simulink model "orion_casestudy_16"  (R2023a)
settings: Solver=VariableStepAuto  StartTime=0.0  StopTime=30  RelTol=1e-3
InitFcn:
  | RandStream.setGlobalStream(RandStream('mt19937ar','seed',sum(100*clock)));
undefined symbols (not defined in the file or in its folder): m, n
(part 3 of 4)

== stateflow chart orion_casestudy_16/DelaySwitch129 ==
  state Operation
  state Sending
  (default) -> Operation : {i=0;}
  (junction 7) -> Operation [order 2]
  Sending -> Operation : after(delay_array(i),msec)
      | {receive(inMsg);outMsg.data=0;send(outMsg);}
  Operation -> (junction 7) : inMsg{i = i + 1;}
  (junction 7) -> Sending [order 1] : [switch_array(i)==0]
  data: switch_array input; delay_array input; outMsg output; inMsg input; i local

== stateflow chart orion_casestudy_16/DelaySwitch130 ==
  state Operation
  state Sending
  (default) -> Operation : {i=0;}
  (junction 7) -> Operation [order 2]
  Sending -> Operation : after(delay_array(i),msec)
      | {receive(inMsg);outMsg.data=0;send(outMsg);}
  Operation -> (junction 7) : inMsg{i = i + 1;}
  (junction 7) -> Sending [order 1] : [switch_array(i)==0]
  data: switch_array input; delay_array input; outMsg output; inMsg input; i local

== stateflow chart orion_casestudy_16/DelaySwitch131 ==
  state Operation
  state Sending
  (default) -> Operation : {i=0;}
  (junction 7) -> Operation [order 2]
  Sending -> Operation : after(delay_array(i),msec)
      | {receive(inMsg);outMsg.data=0;send(outMsg);}
  Operation -> (junction 7) : inMsg{i = i + 1;}
  (junction 7) -> Sending [order 1] : [switch_array(i)==0]
  data: switch_array input; delay_array input; outMsg output; inMsg input; i local

== stateflow chart orion_casestudy_16/DelaySwitch132 ==
  state Operation
  state Sending
  (default) -> Operation : {i=0;}
  (junction 7) -> Operation [order 2]
  Sending -> Operation : after(delay_array(i),msec)
      | {receive(inMsg);outMsg.data=0;send(outMsg);}
  Operation -> (junction 7) : inMsg{i = i + 1;}
  (junction 7) -> Sending [order 1] : [switch_array(i)==0]
  data: switch_array input; delay_array input; outMsg output; inMsg input; i local

== stateflow chart orion_casestudy_16/DelaySwitch133 ==
  state Operation
  state Sending
  (default) -> Operation : {i=0;}
  (junction 7) -> Operation [order 2]
  Sending -> Operation : after(delay_array(i),msec)
      | {receive(inMsg);outMsg.data=0;send(outMsg);}
  Operation -> (junction 7) : inMsg{i = i + 1;}
  (junction 7) -> Sending [order 1] : [switch_array(i)==0]
  data: switch_array input; delay_array input; outMsg output; inMsg input; i local

== stateflow chart orion_casestudy_16/DelaySwitch134 ==
  state Operation
  state Sending
  (default) -> Operation : {i=0;}
  (junction 7) -> Operation [order 2]
  Sending -> Operation : after(delay_array(i),msec)
      | {receive(inMsg);outMsg.data=0;send(outMsg);}
  Operation -> (junction 7) : inMsg{i = i + 1;}
  (junction 7) -> Sending [order 1] : [switch_array(i)==0]
  data: switch_array input; delay_array input; outMsg output; inMsg input; i local

== stateflow chart orion_casestudy_16/DelaySwitch135 ==
  state Operation
  state Sending
  (default) -> Operation : {i=0;}
  (junction 7) -> Operation [order 2]
  Sending -> Operation : after(delay_array(i),msec)
      | {receive(inMsg);outMsg.data=0;send(outMsg);}
  Operation -> (junction 7) : inMsg{i = i + 1;}
  (junction 7) -> Sending [order 1] : [switch_array(i)==0]
  data: switch_array input; delay_array input; outMsg output; inMsg input; i local

== stateflow chart orion_casestudy_16/DelaySwitch136 ==
  state Operation
  state Sending
  (default) -> Operation : {i=0;}
  (junction 7) -> Operation [order 2]
  Sending -> Operation : after(delay_array(i),msec)
      | {receive(inMsg);outMsg.data=0;send(outMsg);}
  Operation -> (junction 7) : inMsg{i = i + 1;}
  (junction 7) -> Sending [order 1] : [switch_array(i)==0]
  data: switch_array input; delay_array input; outMsg output; inMsg input; i local

== stateflow chart orion_casestudy_16/DelaySwitch137 ==
  state Operation
  state Sending
  (default) -> Operation : {i=0;}
  (junction 7) -> Operation [order 2]
  Sending -> Operation : after(delay_array(i),msec)
      | {receive(inMsg);outMsg.data=0;send(outMsg);}
  Operation -> (junction 7) : inMsg{i = i + 1;}
  (junction 7) -> Sending [order 1] : [switch_array(i)==0]
  data: switch_array input; delay_array input; outMsg output; inMsg input; i local

== stateflow chart orion_casestudy_16/DelaySwitch8 ==
  state Operation
  state Sending
  (default) -> Operation : {i=0;}
  (junction 7) -> Operation [order 2]
  Sending -> Operation : after(delay_array(i),msec)
      | {receive(inMsg);outMsg.data=0;send(outMsg);}
  Operation -> (junction 7) : inMsg{i = i + 1;}
  (junction 7) -> Sending [order 1] : [switch_array(i)==0]
  data: switch_array input; delay_array input; outMsg output; inMsg input; i local

== stateflow chart orion_casestudy_16/DelaySwitch138 ==
  state Operation
  state Sending
  (default) -> Operation : {i=0;}
  (junction 7) -> Operation [order 2]
  Sending -> Operation : after(delay_array(i),msec)
      | {receive(inMsg);outMsg.data=0;send(outMsg);}
  Operation -> (junction 7) : inMsg{i = i + 1;}
  (junction 7) -> Sending [order 1] : [switch_array(i)==0]
  data: switch_array input; delay_array input; outMsg output; inMsg input; i local

== stateflow chart orion_casestudy_16/DelaySwitch139 ==
  state Operation
  state Sending
  (default) -> Operation : {i=0;}
  (junction 7) -> Operation [order 2]
  Sending -> Operation : after(delay_array(i),msec)
      | {receive(inMsg);outMsg.data=0;send(outMsg);}
  Operation -> (junction 7) : inMsg{i = i + 1;}
  (junction 7) -> Sending [order 1] : [switch_array(i)==0]
  data: switch_array input; delay_array input; outMsg output; inMsg input; i local

== stateflow chart orion_casestudy_16/DelaySwitch140 ==
  state Operation
  state Sending
  (default) -> Operation : {i=0;}
  (junction 7) -> Operation [order 2]
  Sending -> Operation : after(delay_array(i),msec)
      | {receive(inMsg);outMsg.data=0;send(outMsg);}
  Operation -> (junction 7) : inMsg{i = i + 1;}
  (junction 7) -> Sending [order 1] : [switch_array(i)==0]
  data: switch_array input; delay_array input; outMsg output; inMsg input; i local

== stateflow chart orion_casestudy_16/DelaySwitch141 ==
  state Operation
  state Sending
  (default) -> Operation : {i=0;}
  (junction 7) -> Operation [order 2]
  Sending -> Operation : after(delay_array(i),msec)
      | {receive(inMsg);outMsg.data=0;send(outMsg);}
  Operation -> (junction 7) : inMsg{i = i + 1;}
  (junction 7) -> Sending [order 1] : [switch_array(i)==0]
  data: switch_array input; delay_array input; outMsg output; inMsg input; i local

== stateflow chart orion_casestudy_16/DelaySwitch142 ==
  state Operation
  state Sending
  (default) -> Operation : {i=0;}
  (junction 7) -> Operation [order 2]
  Sending -> Operation : after(delay_array(i),msec)
      | {receive(inMsg);outMsg.data=0;send(outMsg);}
  Operation -> (junction 7) : inMsg{i = i + 1;}
  (junction 7) -> Sending [order 1] : [switch_array(i)==0]
  data: switch_array input; delay_array input; outMsg output; inMsg input; i local

== stateflow chart orion_casestudy_16/DelaySwitch143 ==
  state Operation
  state Sending
  (default) -> Operation : {i=0;}
  (junction 7) -> Operation [order 2]
  Sending -> Operation : after(delay_array(i),msec)
      | {receive(inMsg);outMsg.data=0;send(outMsg);}
  Operation -> (junction 7) : inMsg{i = i + 1;}
  (junction 7) -> Sending [order 1] : [switch_array(i)==0]
  data: switch_array input; delay_array input; outMsg output; inMsg input; i local

== stateflow chart orion_casestudy_16/DelaySwitch144 ==
  state Operation
  state Sending
  (default) -> Operation : {i=0;}
  (junction 7) -> Operation [order 2]
  Sending -> Operation : after(delay_array(i),msec)
      | {receive(inMsg);outMsg.data=0;send(outMsg);}
  Operation -> (junction 7) : inMsg{i = i + 1;}
  (junction 7) -> Sending [order 1] : [switch_array(i)==0]
  data: switch_array input; delay_array input; outMsg output; inMsg input; i local

== stateflow chart orion_casestudy_16/DelaySwitch145 ==
  state Operation
  state Sending
  (default) -> Operation : {i=0;}
  (junction 7) -> Operation [order 2]
  Sending -> Operation : after(delay_array(i),msec)
      | {receive(inMsg);outMsg.data=0;send(outMsg);}
  Operation -> (junction 7) : inMsg{i = i + 1;}
  (junction 7) -> Sending [order 1] : [switch_array(i)==0]
  data: switch_array input; delay_array input; outMsg output; inMsg input; i local

== stateflow chart orion_casestudy_16/DelaySwitch146 ==
  state Operation
  state Sending
  (default) -> Operation : {i=0;}
  (junction 7) -> Operation [order 2]
  Sending -> Operation : after(delay_array(i),msec)
      | {receive(inMsg);outMsg.data=0;send(outMsg);}
  Operation -> (junction 7) : inMsg{i = i + 1;}
  (junction 7) -> Sending [order 1] : [switch_array(i)==0]
  data: switch_array input; delay_array input; outMsg output; inMsg input; i local

== stateflow chart orion_casestudy_16/DelaySwitch147 ==
  state Operation
  state Sending
  (default) -> Operation : {i=0;}
  (junction 7) -> Operation [order 2]
  Sending -> Operation : after(delay_array(i),msec)
      | {receive(inMsg);outMsg.data=0;send(outMsg);}
  Operation -> (junction 7) : inMsg{i = i + 1;}
  (junction 7) -> Sending [order 1] : [switch_array(i)==0]
  data: switch_array input; delay_array input; outMsg output; inMsg input; i local

== stateflow chart orion_casestudy_16/DelaySwitch9 ==
  state Operation
  state Sending
  (default) -> Operation : {i=0;}
  (junction 7) -> Operation [order 2]
  Sending -> Operation : after(delay_array(i),msec)
      | {receive(inMsg);outMsg.data=0;send(outMsg);}
  Operation -> (junction 7) : inMsg{i = i + 1;}
  (junction 7) -> Sending [order 1] : [switch_array(i)==0]
  data: switch_array input; delay_array input; outMsg output; inMsg input; i local

== stateflow chart orion_casestudy_16/DelaySwitch148 ==
  state Operation
  state Sending
  (default) -> Operation : {i=0;}
  (junction 7) -> Operation [order 2]
  Sending -> Operation : after(delay_array(i),msec)
      | {receive(inMsg);outMsg.data=0;send(outMsg);}
  Operation -> (junction 7) : inMsg{i = i + 1;}
  (junction 7) -> Sending [order 1] : [switch_array(i)==0]
  data: switch_array input; delay_array input; outMsg output; inMsg input; i local

== stateflow chart orion_casestudy_16/DelaySwitch149 ==
  state Operation
  state Sending
  (default) -> Operation : {i=0;}
  (junction 7) -> Operation [order 2]
  Sending -> Operation : after(delay_array(i),msec)
      | {receive(inMsg);outMsg.data=0;send(outMsg);}
  Operation -> (junction 7) : inMsg{i = i + 1;}
  (junction 7) -> Sending [order 1] : [switch_array(i)==0]
  data: switch_array input; delay_array input; outMsg output; inMsg input; i local

== stateflow chart orion_casestudy_16/DelaySwitch150 ==
  state Operation
  state Sending
  (default) -> Operation : {i=0;}
  (junction 7) -> Operation [order 2]
  Sending -> Operation : after(delay_array(i),msec)
      | {receive(inMsg);outMsg.data=0;send(outMsg);}
  Operation -> (junction 7) : inMsg{i = i + 1;}
  (junction 7) -> Sending [order 1] : [switch_array(i)==0]
  data: switch_array input; delay_array input; outMsg output; inMsg input; i local

== stateflow chart orion_casestudy_16/DelaySwitch151 ==
  state Operation
  state Sending
  (default) -> Operation : {i=0;}
  (junction 7) -> Operation [order 2]
  Sending -> Operation : after(delay_array(i),msec)
      | {receive(inMsg);outMsg.data=0;send(outMsg);}
  Operation -> (junction 7) : inMsg{i = i + 1;}
  (junction 7) -> Sending [order 1] : [switch_array(i)==0]
  data: switch_array input; delay_array input; outMsg output; inMsg input; i local

== stateflow chart orion_casestudy_16/DelaySwitch152 ==
  state Operation
  state Sending
  (default) -> Operation : {i=0;}
  (junction 7) -> Operation [order 2]
  Sending -> Operation : after(delay_array(i),msec)
      | {receive(inMsg);outMsg.data=0;send(outMsg);}
  Operation -> (junction 7) : inMsg{i = i + 1;}
  (junction 7) -> Sending [order 1] : [switch_array(i)==0]
  data: switch_array input; delay_array input; outMsg output; inMsg input; i local

== stateflow chart orion_casestudy_16/DelaySwitch153 ==
  state Operation
  state Sending
  (default) -> Operation : {i=0;}
  (junction 7) -> Operation [order 2]
  Sending -> Operation : after(delay_array(i),msec)
      | {receive(inMsg);outMsg.data=0;send(outMsg);}
  Operation -> (junction 7) : inMsg{i = i + 1;}
  (junction 7) -> Sending [order 1] : [switch_array(i)==0]
  data: switch_array input; delay_array input; outMsg output; inMsg input; i local

== stateflow chart orion_casestudy_16/DelaySwitch154 ==
  state Operation
  state Sending
  (default) -> Operation : {i=0;}
  (junction 7) -> Operation [order 2]
  Sending -> Operation : after(delay_array(i),msec)
      | {receive(inMsg);outMsg.data=0;send(outMsg);}
  Operation -> (junction 7) : inMsg{i = i + 1;}
  (junction 7) -> Sending [order 1] : [switch_array(i)==0]
  data: switch_array input; delay_array input; outMsg output; inMsg input; i local

== stateflow chart orion_casestudy_16/DelaySwitch155 ==
  state Operation
  state Sending
  (default) -> Operation : {i=0;}
  (junction 7) -> Operation [order 2]
  Sending -> Operation : after(delay_array(i),msec)
      | {receive(inMsg);outMsg.data=0;send(outMsg);}
  Operation -> (junction 7) : inMsg{i = i + 1;}
  (junction 7) -> Sending [order 1] : [switch_array(i)==0]
  data: switch_array input; delay_array input; outMsg output; inMsg input; i local

== stateflow chart orion_casestudy_16/DelaySwitch156 ==
  state Operation
  state Sending
  (default) -> Operation : {i=0;}
  (junction 7) -> Operation [order 2]
  Sending -> Operation : after(delay_array(i),msec)
      | {receive(inMsg);outMsg.data=0;send(outMsg);}
  Operation -> (junction 7) : inMsg{i = i + 1;}
  (junction 7) -> Sending [order 1] : [switch_array(i)==0]
  data: switch_array input; delay_array input; outMsg output; inMsg input; i local

== stateflow chart orion_casestudy_16/DelaySwitch157 ==
  state Operation
  state Sending
  (default) -> Operation : {i=0;}
  (junction 7) -> Operation [order 2]
  Sending -> Operation : after(delay_array(i),msec)
      | {receive(inMsg);outMsg.data=0;send(outMsg);}
  Operation -> (junction 7) : inMsg{i = i + 1;}
  (junction 7) -> Sending [order 1] : [switch_array(i)==0]
  data: switch_array input; delay_array input; outMsg output; inMsg input; i local

== stateflow chart orion_casestudy_16/DelaySwitch10 ==
  state Operation
  state Sending
  (default) -> Operation : {i=0;}
  (junction 7) -> Operation [order 2]
  Sending -> Operation : after(delay_array(i),msec)
      | {receive(inMsg);outMsg.data=0;send(outMsg);}
  Operation -> (junction 7) : inMsg{i = i + 1;}
  (junction 7) -> Sending [order 1] : [switch_array(i)==0]
  data: switch_array input; delay_array input; outMsg output; inMsg input; i local

== stateflow chart orion_casestudy_16/DelaySwitch158 ==
  state Operation
  state Sending
  (default) -> Operation : {i=0;}
  (junction 7) -> Operation [order 2]
  Sending -> Operation : after(delay_array(i),msec)
      | {receive(inMsg);outMsg.data=0;send(outMsg);}
  Operation -> (junction 7) : inMsg{i = i + 1;}
  (junction 7) -> Sending [order 1] : [switch_array(i)==0]
  data: switch_array input; delay_array input; outMsg output; inMsg input; i local

== stateflow chart orion_casestudy_16/DelaySwitch159 ==
  state Operation
  state Sending
  (default) -> Operation : {i=0;}
  (junction 7) -> Operation [order 2]
  Sending -> Operation : after(delay_array(i),msec)
      | {receive(inMsg);outMsg.data=0;send(outMsg);}
  Operation -> (junction 7) : inMsg{i = i + 1;}
  (junction 7) -> Sending [order 1] : [switch_array(i)==0]
  data: switch_array input; delay_array input; outMsg output; inMsg input; i local

== stateflow chart orion_casestudy_16/DelaySwitch160 ==
  state Operation
  state Sending
  (default) -> Operation : {i=0;}
  (junction 7) -> Operation [order 2]
  Sending -> Operation : after(delay_array(i),msec)
      | {receive(inMsg);outMsg.data=0;send(outMsg);}
  Operation -> (junction 7) : inMsg{i = i + 1;}
  (junction 7) -> Sending [order 1] : [switch_array(i)==0]
  data: switch_array input; delay_array input; outMsg output; inMsg input; i local

== stateflow chart orion_casestudy_16/DelaySwitch81 ==
  state Operation
  state Sending
  (default) -> Operation : {i=0;}
  (junction 7) -> Operation [order 2]
  Sending -> Operation : after(delay_array(i),msec)
      | {receive(inMsg);outMsg.data=0;send(outMsg);}
  Operation -> (junction 7) : inMsg{i = i + 1;}
  (junction 7) -> Sending [order 1] : [switch_array(i)==0]
  data: switch_array input; delay_array input; outMsg output; inMsg input; i local

== stateflow chart orion_casestudy_16/DelaySwitch82 ==
  state Operation
  state Sending
  (default) -> Operation : {i=0;}
  (junction 7) -> Operation [order 2]
  Sending -> Operation : after(delay_array(i),msec)
      | {receive(inMsg);outMsg.data=0;send(outMsg);}
  Operation -> (junction 7) : inMsg{i = i + 1;}
  (junction 7) -> Sending [order 1] : [switch_array(i)==0]
  data: switch_array input; delay_array input; outMsg output; inMsg input; i local

== stateflow chart orion_casestudy_16/DelaySwitch83 ==
  state Operation
  state Sending
  (default) -> Operation : {i=0;}
  (junction 7) -> Operation [order 2]
  Sending -> Operation : after(delay_array(i),msec)
      | {receive(inMsg);outMsg.data=0;send(outMsg);}
  Operation -> (junction 7) : inMsg{i = i + 1;}
  (junction 7) -> Sending [order 1] : [switch_array(i)==0]
  data: switch_array input; delay_array input; outMsg output; inMsg input; i local

== stateflow chart orion_casestudy_16/DelaySwitch84 ==
  state Operation
  state Sending
  (default) -> Operation : {i=0;}
  (junction 7) -> Operation [order 2]
  Sending -> Operation : after(delay_array(i),msec)
      | {receive(inMsg);outMsg.data=0;send(outMsg);}
  Operation -> (junction 7) : inMsg{i = i + 1;}
  (junction 7) -> Sending [order 1] : [switch_array(i)==0]
  data: switch_array input; delay_array input; outMsg output; inMsg input; i local

== stateflow chart orion_casestudy_16/DelaySwitch85 ==
  state Operation
  state Sending
  (default) -> Operation : {i=0;}
  (junction 7) -> Operation [order 2]
  Sending -> Operation : after(delay_array(i),msec)
      | {receive(inMsg);outMsg.data=0;send(outMsg);}
  Operation -> (junction 7) : inMsg{i = i + 1;}
  (junction 7) -> Sending [order 1] : [switch_array(i)==0]
  data: switch_array input; delay_array input; outMsg output; inMsg input; i local

== stateflow chart orion_casestudy_16/DelaySwitch86 ==
  state Operation
  state Sending
  (default) -> Operation : {i=0;}
  (junction 7) -> Operation [order 2]
  Sending -> Operation : after(delay_array(i),msec)
      | {receive(inMsg);outMsg.data=0;send(outMsg);}
  Operation -> (junction 7) : inMsg{i = i + 1;}
  (junction 7) -> Sending [order 1] : [switch_array(i)==0]
  data: switch_array input; delay_array input; outMsg output; inMsg input; i local

== stateflow chart orion_casestudy_16/DelaySwitch87 ==
  state Operation
  state Sending
  (default) -> Operation : {i=0;}
  (junction 7) -> Operation [order 2]
  Sending -> Operation : after(delay_array(i),msec)
      | {receive(inMsg);outMsg.data=0;send(outMsg);}
  Operation -> (junction 7) : inMsg{i = i + 1;}
  (junction 7) -> Sending [order 1] : [switch_array(i)==0]
  data: switch_array input; delay_array input; outMsg output; inMsg input; i local

== stateflow chart orion_casestudy_16/OverallState ==
  settings: updateMethod=CONTINUOUS
  state NotConnected
    op_time=temporalCount(msec);
  state Connected
    entry:
    connStatus=1;
  (default) -> NotConnected : {connStatus=0;
      | op_time=0;}
  NotConnected -> Connected : [(conn1==2 && conn2==2) ||  (conn3==2 && conn4==2) ||  (conn5==2 && conn6==2) ||  (conn7==2 && conn8==2) ||  (conn9==2 && conn10==2) ||  (conn11==2 && conn12==2) ||  (conn13==2 && conn14==2) ||  (conn15==2 && conn16==2) || (conn17==2 && conn18==2) ||  (conn19==2 && conn20==2) ||  (conn21==2 && conn22==2) ||  (conn23==2 && conn24==2) ||  (conn25==2 && conn26==2) ||  (conn27==2 && conn28==2) ||  (conn29==2 && conn30==2) ||  (conn31==2 && conn32==2)]
  data: conn32 input; conn26 input; conn23 input; conn1 input; conn2 input; connStatus output; op_time output; conn3 input; conn4 input; conn5 input; conn6 input; conn7 input; conn8 input; conn9 input; conn10 input; conn11 input; conn12 input; conn13 input; conn14 input; conn15 input; conn16 input; conn17 input; conn18 input; conn19 input; conn20 input; conn21 input; conn22 input; conn24 input; conn25 input; conn27 input; conn28 input; conn29 input; conn30 input; conn31 input

== stateflow chart orion_casestudy_16/DelaySwitch88 ==
  state Operation
  state Sending
  (default) -> Operation : {i=0;}
  (junction 7) -> Operation [order 2]
  Sending -> Operation : after(delay_array(i),msec)
      | {receive(inMsg);outMsg.data=0;send(outMsg);}
  Operation -> (junction 7) : inMsg{i = i + 1;}
  (junction 7) -> Sending [order 1] : [switch_array(i)==0]
  data: switch_array input; delay_array input; outMsg output; inMsg input; i local

== stateflow chart orion_casestudy_16/DelaySwitch89 ==
  state Operation
  state Sending
  (default) -> Operation : {i=0;}
  (junction 7) -> Operation [order 2]
  Sending -> Operation : after(delay_array(i),msec)
      | {receive(inMsg);outMsg.data=0;send(outMsg);}
  Operation -> (junction 7) : inMsg{i = i + 1;}
  (junction 7) -> Sending [order 1] : [switch_array(i)==0]
  data: switch_array input; delay_array input; outMsg output; inMsg input; i local

== stateflow chart orion_casestudy_16/DelaySwitch90 ==
  state Operation
  state Sending
  (default) -> Operation : {i=0;}
  (junction 7) -> Operation [order 2]
  Sending -> Operation : after(delay_array(i),msec)
      | {receive(inMsg);outMsg.data=0;send(outMsg);}
  Operation -> (junction 7) : inMsg{i = i + 1;}
  (junction 7) -> Sending [order 1] : [switch_array(i)==0]
  data: switch_array input; delay_array input; outMsg output; inMsg input; i local

== stateflow chart orion_casestudy_16/DelaySwitch91 ==
  state Operation
  state Sending
  (default) -> Operation : {i=0;}
  (junction 7) -> Operation [order 2]
  Sending -> Operation : after(delay_array(i),msec)
      | {receive(inMsg);outMsg.data=0;send(outMsg);}
  Operation -> (junction 7) : inMsg{i = i + 1;}
  (junction 7) -> Sending [order 1] : [switch_array(i)==0]
  data: switch_array input; delay_array input; outMsg output; inMsg input; i local

== stateflow chart orion_casestudy_16/DelaySwitch92 ==
  state Operation
  state Sending
  (default) -> Operation : {i=0;}
  (junction 7) -> Operation [order 2]
  Sending -> Operation : after(delay_array(i),msec)
      | {receive(inMsg);outMsg.data=0;send(outMsg);}
  Operation -> (junction 7) : inMsg{i = i + 1;}
  (junction 7) -> Sending [order 1] : [switch_array(i)==0]
  data: switch_array input; delay_array input; outMsg output; inMsg input; i local

== stateflow chart orion_casestudy_16/DelaySwitch93 ==
  state Operation
  state Sending
  (default) -> Operation : {i=0;}
  (junction 7) -> Operation [order 2]
  Sending -> Operation : after(delay_array(i),msec)
      | {receive(inMsg);outMsg.data=0;send(outMsg);}
  Operation -> (junction 7) : inMsg{i = i + 1;}
  (junction 7) -> Sending [order 1] : [switch_array(i)==0]
  data: switch_array input; delay_array input; outMsg output; inMsg input; i local

== stateflow chart orion_casestudy_16/DelaySwitch94 ==
  state Operation
  state Sending
  (default) -> Operation : {i=0;}
  (junction 7) -> Operation [order 2]
  Sending -> Operation : after(delay_array(i),msec)
      | {receive(inMsg);outMsg.data=0;send(outMsg);}
  Operation -> (junction 7) : inMsg{i = i + 1;}
  (junction 7) -> Sending [order 1] : [switch_array(i)==0]
  data: switch_array input; delay_array input; outMsg output; inMsg input; i local

== stateflow chart orion_casestudy_16/DelaySwitch95 ==
  state Operation
  state Sending
  (default) -> Operation : {i=0;}
  (junction 7) -> Operation [order 2]
  Sending -> Operation : after(delay_array(i),msec)
      | {receive(inMsg);outMsg.data=0;send(outMsg);}
  Operation -> (junction 7) : inMsg{i = i + 1;}
  (junction 7) -> Sending [order 1] : [switch_array(i)==0]
  data: switch_array input; delay_array input; outMsg output; inMsg input; i local

== stateflow chart orion_casestudy_16/DelaySwitch96 ==
  state Operation
  state Sending
  (default) -> Operation : {i=0;}
  (junction 7) -> Operation [order 2]
  Sending -> Operation : after(delay_array(i),msec)
      | {receive(inMsg);outMsg.data=0;send(outMsg);}
  Operation -> (junction 7) : inMsg{i = i + 1;}
  (junction 7) -> Sending [order 1] : [switch_array(i)==0]
  data: switch_array input; delay_array input; outMsg output; inMsg input; i local

== stateflow chart orion_casestudy_16/DelaySwitch97 ==
  state Operation
  state Sending
  (default) -> Operation : {i=0;}
  (junction 7) -> Operation [order 2]
  Sending -> Operation : after(delay_array(i),msec)
      | {receive(inMsg);outMsg.data=0;send(outMsg);}
  Operation -> (junction 7) : inMsg{i = i + 1;}
  (junction 7) -> Sending [order 1] : [switch_array(i)==0]
  data: switch_array input; delay_array input; outMsg output; inMsg input; i local

== stateflow chart orion_casestudy_16/DelaySwitch98 ==
  state Operation
  state Sending
  (default) -> Operation : {i=0;}
  (junction 7) -> Operation [order 2]
  Sending -> Operation : after(delay_array(i),msec)
      | {receive(inMsg);outMsg.data=0;send(outMsg);}
  Operation -> (junction 7) : inMsg{i = i + 1;}
  (junction 7) -> Sending [order 1] : [switch_array(i)==0]
  data: switch_array input; delay_array input; outMsg output; inMsg input; i local

== stateflow chart orion_casestudy_16/DelaySwitch99 ==
  state Operation
  state Sending
  (default) -> Operation : {i=0;}
  (junction 7) -> Operation [order 2]
  Sending -> Operation : after(delay_array(i),msec)
      | {receive(inMsg);outMsg.data=0;send(outMsg);}
  Operation -> (junction 7) : inMsg{i = i + 1;}
  (junction 7) -> Sending [order 1] : [switch_array(i)==0]
  data: switch_array input; delay_array input; outMsg output; inMsg input; i local

== stateflow chart orion_casestudy_16/Master10 ==
  settings: updateMethod=CONTINUOUS
  state Connected
    entry:
    connStatus=2;
    state KeepAliveSendTimeout [parallel]
      settings: executionOrder=1
      state KeepAliveSend
      (default) -> KeepAliveSend
      KeepAliveSend -> KeepAliveSend [order 1] : after(delay_array(i)*5,msec)
          | {OrionKeepAliveOut.data=0;
          | send(OrionKeepAliveOut);
          | i = i + 1;}
      KeepAliveSend -> KeepAliveSend [order 2] : SendDataIn
          | {OrionAppDataOut.data=0;
          | send(OrionAppDataOut);}
    state KeepAliveRecieveTimeout [parallel]
      settings: executionOrder=2
      state KeepAlineRec
      (default) -> KeepAlineRec
      KeepAlineRec -> KeepAlineRec [order 2] : OrionKeepAliveIn
      KeepAlineRec -> KeepAlineRec [order 3] : OrionAppDataIn
  state Closed
    entry:
    connStatus=0;
  state Connecting
    entry:
    connStatus=1;
  Connected -> (junction 6) [order 1] : OrionConnConfIn
  (default) -> Closed : {i=1;}
  Connected -> (junction 6) [order 2] : OrionConnRespIn
  Connected -> (junction 6) [order 3] : OrionConnReqIn
  (junction 6) -> Closed
  KeepAlineRec -> Closed [order 1] : after(delay_array(i)*5,msec)
      | {i = i + 1;}
  Connecting -> (junction 36) [order 5] : OrionConnReqIn
  (junction 36) -> Closed
  Connecting -> (junction 36) [order 4] : OrionConnRespIn
  Connecting -> (junction 36) [order 2] : OrionKeepAliveIn
  Connecting -> Closed [order 3] : after(delay_array(i)*5,msec)
      | {i = i + 1;}
  Closed -> Connecting [order 2] : after(delay_array(i)*5,msec)
      | {OrionConnReqOut.data=0;send(OrionConnReqOut);i = i + 1;}
  Closed -> Connecting [order 1] : OrionConnReqIn
      | {OrionConnRespOut.data=0;send(OrionConnRespOut);}
  Connecting -> Connected [order 1] : OrionConnRespIn
      | {OrionConnConfOut.data=0;
      | send(OrionConnConfOut);}
  data: delay_array input; OrionKeepAliveOut output; OrionKeepAliveIn input; OrionConnConfOut output; OrionConnConfIn input; OrionConnRespOut output; OrionAppDataOut output; OrionAppDataIn input; OrionConnRespIn input; OrionConnReqIn input; OrionConnReqOut output; connStatus output; SendDataIn local; i local

== stateflow chart orion_casestudy_16/Master11 ==
  settings: updateMethod=CONTINUOUS
  state Connected
    entry:
    connStatus=2;
    state KeepAliveSendTimeout [parallel]
      settings: executionOrder=1
      state KeepAliveSend
      (default) -> KeepAliveSend
      KeepAliveSend -> KeepAliveSend [order 1] : after(delay_array(i)*5,msec)
          | {OrionKeepAliveOut.data=0;
          | send(OrionKeepAliveOut);
          | i = i + 1;}
      KeepAliveSend -> KeepAliveSend [order 2] : SendDataIn
          | {OrionAppDataOut.data=0;
          | send(OrionAppDataOut);}
    state KeepAliveRecieveTimeout [parallel]
      settings: executionOrder=2
      state KeepAlineRec
      (default) -> KeepAlineRec
      KeepAlineRec -> KeepAlineRec [order 2] : OrionKeepAliveIn
      KeepAlineRec -> KeepAlineRec [order 3] : OrionAppDataIn
  state Closed
    entry:
    connStatus=0;
  state Connecting
    entry:
    connStatus=1;
  Connected -> (junction 6) [order 1] : OrionConnConfIn
  (default) -> Closed : {i=1;}
  Connected -> (junction 6) [order 2] : OrionConnRespIn
  Connected -> (junction 6) [order 3] : OrionConnReqIn
  (junction 6) -> Closed
  KeepAlineRec -> Closed [order 1] : after(delay_array(i)*5,msec)
      | {i = i + 1;}
  Connecting -> (junction 36) [order 5] : OrionConnReqIn
  (junction 36) -> Closed
  Connecting -> (junction 36) [order 4] : OrionConnRespIn
  Connecting -> (junction 36) [order 2] : OrionKeepAliveIn
  Connecting -> Closed [order 3] : after(delay_array(i)*5,msec)
      | {i = i + 1;}
  Closed -> Connecting [order 2] : after(delay_array(i)*5,msec)
      | {OrionConnReqOut.data=0;send(OrionConnReqOut);i = i + 1;}
  Closed -> Connecting [order 1] : OrionConnReqIn
      | {OrionConnRespOut.data=0;send(OrionConnRespOut);}
  Connecting -> Connected [order 1] : OrionConnRespIn
      | {OrionConnConfOut.data=0;
      | send(OrionConnConfOut);}
  data: delay_array input; OrionKeepAliveOut output; OrionKeepAliveIn input; OrionConnConfOut output; OrionConnConfIn input; OrionConnRespOut output; OrionAppDataOut output; OrionAppDataIn input; OrionConnRespIn input; OrionConnReqIn input; OrionConnReqOut output; connStatus output; SendDataIn local; i local

== stateflow chart orion_casestudy_16/Master12 ==
  settings: updateMethod=CONTINUOUS
  state Connected
    entry:
    connStatus=2;
    state KeepAliveSendTimeout [parallel]
      settings: executionOrder=1
      state KeepAliveSend
      (default) -> KeepAliveSend
      KeepAliveSend -> KeepAliveSend [order 1] : after(delay_array(i)*5,msec)
          | {OrionKeepAliveOut.data=0;
          | send(OrionKeepAliveOut);
          | i = i + 1;}
      KeepAliveSend -> KeepAliveSend [order 2] : SendDataIn
          | {OrionAppDataOut.data=0;
          | send(OrionAppDataOut);}
    state KeepAliveRecieveTimeout [parallel]
      settings: executionOrder=2
      state KeepAlineRec
      (default) -> KeepAlineRec
      KeepAlineRec -> KeepAlineRec [order 2] : OrionKeepAliveIn
      KeepAlineRec -> KeepAlineRec [order 3] : OrionAppDataIn
  state Closed
    entry:
    connStatus=0;
  state Connecting
    entry:
    connStatus=1;
  Connected -> (junction 6) [order 1] : OrionConnConfIn
  (default) -> Closed : {i=1;}
  Connected -> (junction 6) [order 2] : OrionConnRespIn
  Connected -> (junction 6) [order 3] : OrionConnReqIn
  (junction 6) -> Closed
  KeepAlineRec -> Closed [order 1] : after(delay_array(i)*5,msec)
      | {i = i + 1;}
  Connecting -> (junction 36) [order 5] : OrionConnReqIn
  (junction 36) -> Closed
  Connecting -> (junction 36) [order 4] : OrionConnRespIn
  Connecting -> (junction 36) [order 2] : OrionKeepAliveIn
  Connecting -> Closed [order 3] : after(delay_array(i)*5,msec)
      | {i = i + 1;}
  Closed -> Connecting [order 2] : after(delay_array(i)*5,msec)
      | {OrionConnReqOut.data=0;send(OrionConnReqOut);i = i + 1;}
  Closed -> Connecting [order 1] : OrionConnReqIn
      | {OrionConnRespOut.data=0;send(OrionConnRespOut);}
  Connecting -> Connected [order 1] : OrionConnRespIn
      | {OrionConnConfOut.data=0;
      | send(OrionConnConfOut);}
  data: delay_array input; OrionKeepAliveOut output; OrionKeepAliveIn input; OrionConnConfOut output; OrionConnConfIn input; OrionConnRespOut output; OrionAppDataOut output; OrionAppDataIn input; OrionConnRespIn input; OrionConnReqIn input; OrionConnReqOut output; connStatus output; SendDataIn local; i local

== stateflow chart orion_casestudy_16/Master13 ==
  settings: updateMethod=CONTINUOUS
  state Connected
    entry:
    connStatus=2;
    state KeepAliveSendTimeout [parallel]
      settings: executionOrder=1
      state KeepAliveSend
      (default) -> KeepAliveSend
      KeepAliveSend -> KeepAliveSend [order 1] : after(delay_array(i)*5,msec)
          | {OrionKeepAliveOut.data=0;
          | send(OrionKeepAliveOut);
          | i = i + 1;}
      KeepAliveSend -> KeepAliveSend [order 2] : SendDataIn
          | {OrionAppDataOut.data=0;
          | send(OrionAppDataOut);}
    state KeepAliveRecieveTimeout [parallel]
      settings: executionOrder=2
      state KeepAlineRec
      (default) -> KeepAlineRec
      KeepAlineRec -> KeepAlineRec [order 2] : OrionKeepAliveIn
      KeepAlineRec -> KeepAlineRec [order 3] : OrionAppDataIn
  state Closed
    entry:
    connStatus=0;
  state Connecting
    entry:
    connStatus=1;
  Connected -> (junction 6) [order 1] : OrionConnConfIn
  (default) -> Closed : {i=1;}
  Connected -> (junction 6) [order 2] : OrionConnRespIn
  Connected -> (junction 6) [order 3] : OrionConnReqIn
  (junction 6) -> Closed
  KeepAlineRec -> Closed [order 1] : after(delay_array(i)*5,msec)
      | {i = i + 1;}
  Connecting -> (junction 36) [order 5] : OrionConnReqIn
  (junction 36) -> Closed
  Connecting -> (junction 36) [order 4] : OrionConnRespIn
  Connecting -> (junction 36) [order 2] : OrionKeepAliveIn
  Connecting -> Closed [order 3] : after(delay_array(i)*5,msec)
      | {i = i + 1;}
  Closed -> Connecting [order 2] : after(delay_array(i)*5,msec)
      | {OrionConnReqOut.data=0;send(OrionConnReqOut);i = i + 1;}
  Closed -> Connecting [order 1] : OrionConnReqIn
      | {OrionConnRespOut.data=0;send(OrionConnRespOut);}
  Connecting -> Connected [order 1] : OrionConnRespIn
      | {OrionConnConfOut.data=0;
      | send(OrionConnConfOut);}
  data: delay_array input; OrionKeepAliveOut output; OrionKeepAliveIn input; OrionConnConfOut output; OrionConnConfIn input; OrionConnRespOut output; OrionAppDataOut output; OrionAppDataIn input; OrionConnRespIn input; OrionConnReqIn input; OrionConnReqOut output; connStatus output; SendDataIn local; i local

== stateflow chart orion_casestudy_16/Master14 ==
  settings: updateMethod=CONTINUOUS
  state Connected
    entry:
    connStatus=2;
    state KeepAliveSendTimeout [parallel]
      settings: executionOrder=1
      state KeepAliveSend
      (default) -> KeepAliveSend
      KeepAliveSend -> KeepAliveSend [order 1] : after(delay_array(i)*5,msec)
          | {OrionKeepAliveOut.data=0;
          | send(OrionKeepAliveOut);
          | i = i + 1;}
      KeepAliveSend -> KeepAliveSend [order 2] : SendDataIn
          | {OrionAppDataOut.data=0;
          | send(OrionAppDataOut);}
    state KeepAliveRecieveTimeout [parallel]
      settings: executionOrder=2
      state KeepAlineRec
      (default) -> KeepAlineRec
      KeepAlineRec -> KeepAlineRec [order 2] : OrionKeepAliveIn
      KeepAlineRec -> KeepAlineRec [order 3] : OrionAppDataIn
  state Closed
    entry:
    connStatus=0;
  state Connecting
    entry:
    connStatus=1;
  Connected -> (junction 6) [order 1] : OrionConnConfIn
  (default) -> Closed : {i=1;}
  Connected -> (junction 6) [order 2] : OrionConnRespIn
  Connected -> (junction 6) [order 3] : OrionConnReqIn
  (junction 6) -> Closed
  KeepAlineRec -> Closed [order 1] : after(delay_array(i)*5,msec)
      | {i = i + 1;}
  Connecting -> (junction 36) [order 5] : OrionConnReqIn
  (junction 36) -> Closed
  Connecting -> (junction 36) [order 4] : OrionConnRespIn
  Connecting -> (junction 36) [order 2] : OrionKeepAliveIn
  Connecting -> Closed [order 3] : after(delay_array(i)*5,msec)
      | {i = i + 1;}
  Closed -> Connecting [order 2] : after(delay_array(i)*5,msec)
      | {OrionConnReqOut.data=0;send(OrionConnReqOut);i = i + 1;}
  Closed -> Connecting [order 1] : OrionConnReqIn
      | {OrionConnRespOut.data=0;send(OrionConnRespOut);}
  Connecting -> Connected [order 1] : OrionConnRespIn
      | {OrionConnConfOut.data=0;
      | send(OrionConnConfOut);}
  data: delay_array input; OrionKeepAliveOut output; OrionKeepAliveIn input; OrionConnConfOut output; OrionConnConfIn input; OrionConnRespOut output; OrionAppDataOut output; OrionAppDataIn input; OrionConnRespIn input; OrionConnReqIn input; OrionConnReqOut output; connStatus output; SendDataIn local; i local

== stateflow chart orion_casestudy_16/DelaySwitch11 ==
  state Operation
  state Sending
  (default) -> Operation : {i=0;}
  (junction 7) -> Operation [order 2]
  Sending -> Operation : after(delay_array(i),msec)
      | {receive(inMsg);outMsg.data=0;send(outMsg);}
  Operation -> (junction 7) : inMsg{i = i + 1;}
  (junction 7) -> Sending [order 1] : [switch_array(i)==0]
  data: switch_array input; delay_array input; outMsg output; inMsg input; i local

== stateflow chart orion_casestudy_16/Master15 ==
  settings: updateMethod=CONTINUOUS
  state Connected
    entry:
    connStatus=2;
    state KeepAliveSendTimeout [parallel]
      settings: executionOrder=1
      state KeepAliveSend
      (default) -> KeepAliveSend
      KeepAliveSend -> KeepAliveSend [order 1] : after(delay_array(i)*5,msec)
          | {OrionKeepAliveOut.data=0;
          | send(OrionKeepAliveOut);
          | i = i + 1;}
      KeepAliveSend -> KeepAliveSend [order 2] : SendDataIn
          | {OrionAppDataOut.data=0;
          | send(OrionAppDataOut);}
    state KeepAliveRecieveTimeout [parallel]
      settings: executionOrder=2
      state KeepAlineRec
      (default) -> KeepAlineRec
      KeepAlineRec -> KeepAlineRec [order 2] : OrionKeepAliveIn
      KeepAlineRec -> KeepAlineRec [order 3] : OrionAppDataIn
  state Closed
    entry:
    connStatus=0;
  state Connecting
    entry:
    connStatus=1;
  Connected -> (junction 6) [order 1] : OrionConnConfIn
  (default) -> Closed : {i=1;}
  Connected -> (junction 6) [order 2] : OrionConnRespIn
  Connected -> (junction 6) [order 3] : OrionConnReqIn
  (junction 6) -> Closed
  KeepAlineRec -> Closed [order 1] : after(delay_array(i)*5,msec)
      | {i = i + 1;}
  Connecting -> (junction 36) [order 5] : OrionConnReqIn
  (junction 36) -> Closed
  Connecting -> (junction 36) [order 4] : OrionConnRespIn
  Connecting -> (junction 36) [order 2] : OrionKeepAliveIn
  Connecting -> Closed [order 3] : after(delay_array(i)*5,msec)
      | {i = i + 1;}
  Closed -> Connecting [order 2] : after(delay_array(i)*5,msec)
      | {OrionConnReqOut.data=0;send(OrionConnReqOut);i = i + 1;}
  Closed -> Connecting [order 1] : OrionConnReqIn
      | {OrionConnRespOut.data=0;send(OrionConnRespOut);}
  Connecting -> Connected [order 1] : OrionConnRespIn
      | {OrionConnConfOut.data=0;
      | send(OrionConnConfOut);}
  data: delay_array input; OrionKeepAliveOut output; OrionKeepAliveIn input; OrionConnConfOut output; OrionConnConfIn input; OrionConnRespOut output; OrionAppDataOut output; OrionAppDataIn input; OrionConnRespIn input; OrionConnReqIn input; OrionConnReqOut output; connStatus output; SendDataIn local; i local

== stateflow chart orion_casestudy_16/Master8 ==
  settings: updateMethod=CONTINUOUS
  state Connected
    entry:
    connStatus=2;
    state KeepAliveSendTimeout [parallel]
      settings: executionOrder=1
      state KeepAliveSend
      (default) -> KeepAliveSend
      KeepAliveSend -> KeepAliveSend [order 1] : after(delay_array(i)*5,msec)
          | {OrionKeepAliveOut.data=0;
          | send(OrionKeepAliveOut);
          | i = i + 1;}
      KeepAliveSend -> KeepAliveSend [order 2] : SendDataIn
          | {OrionAppDataOut.data=0;
          | send(OrionAppDataOut);}
    state KeepAliveRecieveTimeout [parallel]
      settings: executionOrder=2
      state KeepAlineRec
      (default) -> KeepAlineRec
      KeepAlineRec -> KeepAlineRec [order 2] : OrionKeepAliveIn
      KeepAlineRec -> KeepAlineRec [order 3] : OrionAppDataIn
  state Closed
    entry:
    connStatus=0;
  state Connecting
    entry:
    connStatus=1;
  Connected -> (junction 6) [order 1] : OrionConnConfIn
  (default) -> Closed : {i=1;}
  Connected -> (junction 6) [order 2] : OrionConnRespIn
  Connected -> (junction 6) [order 3] : OrionConnReqIn
  (junction 6) -> Closed
  KeepAlineRec -> Closed [order 1] : after(delay_array(i)*5,msec)
      | {i = i + 1;}
  Connecting -> (junction 36) [order 5] : OrionConnReqIn
  (junction 36) -> Closed
  Connecting -> (junction 36) [order 4] : OrionConnRespIn
  Connecting -> (junction 36) [order 2] : OrionKeepAliveIn
  Connecting -> Closed [order 3] : after(delay_array(i)*5,msec)
      | {i = i + 1;}
  Closed -> Connecting [order 2] : after(delay_array(i)*5,msec)
      | {OrionConnReqOut.data=0;send(OrionConnReqOut);i = i + 1;}
  Closed -> Connecting [order 1] : OrionConnReqIn
      | {OrionConnRespOut.data=0;send(OrionConnRespOut);}
  Connecting -> Connected [order 1] : OrionConnRespIn
      | {OrionConnConfOut.data=0;
      | send(OrionConnConfOut);}
  data: delay_array input; OrionKeepAliveOut output; OrionKeepAliveIn input; OrionConnConfOut output; OrionConnConfIn input; OrionConnRespOut output; OrionAppDataOut output; OrionAppDataIn input; OrionConnRespIn input; OrionConnReqIn input; OrionConnReqOut output; connStatus output; SendDataIn local; i local

== stateflow chart orion_casestudy_16/Master9 ==
  settings: updateMethod=CONTINUOUS
  state Connected
    entry:
    connStatus=2;
    state KeepAliveSendTimeout [parallel]
      settings: executionOrder=1
      state KeepAliveSend
      (default) -> KeepAliveSend
      KeepAliveSend -> KeepAliveSend [order 1] : after(delay_array(i)*5,msec)
          | {OrionKeepAliveOut.data=0;
          | send(OrionKeepAliveOut);
          | i = i + 1;}
      KeepAliveSend -> KeepAliveSend [order 2] : SendDataIn
          | {OrionAppDataOut.data=0;
          | send(OrionAppDataOut);}
    state KeepAliveRecieveTimeout [parallel]
      settings: executionOrder=2
      state KeepAlineRec
      (default) -> KeepAlineRec
      KeepAlineRec -> KeepAlineRec [order 2] : OrionKeepAliveIn
      KeepAlineRec -> KeepAlineRec [order 3] : OrionAppDataIn
  state Closed
    entry:
    connStatus=0;
  state Connecting
    entry:
    connStatus=1;
  Connected -> (junction 6) [order 1] : OrionConnConfIn
  (default) -> Closed : {i=1;}
  Connected -> (junction 6) [order 2] : OrionConnRespIn
  Connected -> (junction 6) [order 3] : OrionConnReqIn
  (junction 6) -> Closed
  KeepAlineRec -> Closed [order 1] : after(delay_array(i)*5,msec)
      | {i = i + 1;}
  Connecting -> (junction 36) [order 5] : OrionConnReqIn
  (junction 36) -> Closed
  Connecting -> (junction 36) [order 4] : OrionConnRespIn
  Connecting -> (junction 36) [order 2] : OrionKeepAliveIn
  Connecting -> Closed [order 3] : after(delay_array(i)*5,msec)
      | {i = i + 1;}
  Closed -> Connecting [order 2] : after(delay_array(i)*5,msec)
      | {OrionConnReqOut.data=0;send(OrionConnReqOut);i = i + 1;}
  Closed -> Connecting [order 1] : OrionConnReqIn
      | {OrionConnRespOut.data=0;send(OrionConnRespOut);}
  Connecting -> Connected [order 1] : OrionConnRespIn
      | {OrionConnConfOut.data=0;
      | send(OrionConnConfOut);}
  data: delay_array input; OrionKeepAliveOut output; OrionKeepAliveIn input; OrionConnConfOut output; OrionConnConfIn input; OrionConnRespOut output; OrionAppDataOut output; OrionAppDataIn input; OrionConnRespIn input; OrionConnReqIn input; OrionConnReqOut output; connStatus output; SendDataIn local; i local

== stateflow chart orion_casestudy_16/DelaySwitch12 ==
  state Operation
  state Sending
  (default) -> Operation : {i=0;}
  (junction 7) -> Operation [order 2]
  Sending -> Operation : after(delay_array(i),msec)
      | {receive(inMsg);outMsg.data=0;send(outMsg);}
  Operation -> (junction 7) : inMsg{i = i + 1;}
  (junction 7) -> Sending [order 1] : [switch_array(i)==0]
  data: switch_array input; delay_array input; outMsg output; inMsg input; i local

== stateflow chart orion_casestudy_16/Slave10 ==
  settings: updateMethod=CONTINUOUS
  state Connected
    entry:
    connStatus=2;
    state KeepAliveSendTimeout [parallel]
      settings: executionOrder=1
      state KeepAliveSend
      (default) -> KeepAliveSend
      KeepAliveSend -> KeepAliveSend [order 1] : after(delay_array(i)*5,msec)
          |  {OrionKeepAliveOut.data=0;
          | send(OrionKeepAliveOut);i = i + 1;}
      KeepAliveSend -> KeepAliveSend [order 2] : SendDataIn
          | {OrionAppDataOut.data=0;
          | send(OrionAppDataOut);}
    state KeepAliveRecieveTimeout [parallel]
      settings: executionOrder=2
      state KeepAlineRec
      (default) -> KeepAlineRec
      KeepAlineRec -> KeepAlineRec [order 2] : OrionKeepAliveIn
      KeepAlineRec -> KeepAlineRec [order 3] : OrionAppDataIn
  state Closed
    entry:
    connStatus=0;
  state Connecting
    entry:
    connStatus=1;
  Connected -> (junction 6) [order 2] : OrionConnRespIn
  Connected -> (junction 6) [order 3] : OrionConnReqIn
  (default) -> Closed : {i=1;}
  (junction 6) -> Closed
  Connected -> (junction 6) [order 1] : OrionConnConfIn
  KeepAlineRec -> Closed [order 1] : after(delay_array(i)*5,msec)
      | {i = i + 1;}
  Connecting -> (junction 36) [order 6] : OrionAppDataIn
  Connecting -> (junction 36) [order 5] : OrionConnReqIn
  (junction 36) -> Closed
  Connecting -> (junction 36) [order 4] : OrionConnRespIn
  Connecting -> (junction 36) [order 3] : OrionKeepAliveIn
  Closed -> Connecting : OrionConnReqIn
      | {OrionConnRespOut.data=0;
      | send(OrionConnRespOut);}
  Connecting -> Closed [order 1] : after(delay_array(i)*5,msec)
      | {i = i + 1;}
  Connecting -> Connected [order 2] : OrionConnConfIn{OrionConnConfOut.data=0;send(OrionConnConfOut);}
  data: OrionKeepAliveIn input; OrionConnConfOut output; OrionConnRespOut output; OrionKeepAliveOut output; OrionAppDataOut output; OrionAppDataIn input; OrionConnRespIn input; OrionConnReqIn input; OrionConnReqOut output size=1; connStatus output; SendDataIn local; OrionConnConfIn input; delay_array input; i local

== stateflow chart orion_casestudy_16/Slave11 ==
  settings: updateMethod=CONTINUOUS
  state Connected
    entry:
    connStatus=2;
    state KeepAliveSendTimeout [parallel]
      settings: executionOrder=1
      state KeepAliveSend
      (default) -> KeepAliveSend
      KeepAliveSend -> KeepAliveSend [order 1] : after(delay_array(i)*5,msec)
          |  {OrionKeepAliveOut.data=0;
          | send(OrionKeepAliveOut);i = i + 1;}
      KeepAliveSend -> KeepAliveSend [order 2] : SendDataIn
          | {OrionAppDataOut.data=0;
          | send(OrionAppDataOut);}
    state KeepAliveRecieveTimeout [parallel]
      settings: executionOrder=2
      state KeepAlineRec
      (default) -> KeepAlineRec
      KeepAlineRec -> KeepAlineRec [order 2] : OrionKeepAliveIn
      KeepAlineRec -> KeepAlineRec [order 3] : OrionAppDataIn
  state Closed
    entry:
    connStatus=0;
  state Connecting
    entry:
    connStatus=1;
  Connected -> (junction 6) [order 2] : OrionConnRespIn
  Connected -> (junction 6) [order 3] : OrionConnReqIn
  (default) -> Closed : {i=1;}
  (junction 6) -> Closed
  Connected -> (junction 6) [order 1] : OrionConnConfIn
  KeepAlineRec -> Closed [order 1] : after(delay_array(i)*5,msec)
      | {i = i + 1;}
  Connecting -> (junction 36) [order 6] : OrionAppDataIn
  Connecting -> (junction 36) [order 5] : OrionConnReqIn
  (junction 36) -> Closed
  Connecting -> (junction 36) [order 4] : OrionConnRespIn
  Connecting -> (junction 36) [order 3] : OrionKeepAliveIn
  Closed -> Connecting : OrionConnReqIn
      | {OrionConnRespOut.data=0;
      | send(OrionConnRespOut);}
  Connecting -> Closed [order 1] : after(delay_array(i)*5,msec)
      | {i = i + 1;}
  Connecting -> Connected [order 2] : OrionConnConfIn{OrionConnConfOut.data=0;send(OrionConnConfOut);}
  data: OrionKeepAliveIn input; OrionConnConfOut output; OrionConnRespOut output; OrionKeepAliveOut output; OrionAppDataOut output; OrionAppDataIn input; OrionConnRespIn input; OrionConnReqIn input; OrionConnReqOut output size=1; connStatus output; SendDataIn local; OrionConnConfIn input; delay_array input; i local

== stateflow chart orion_casestudy_16/Slave12 ==
  settings: updateMethod=CONTINUOUS
  state Connected
    entry:
    connStatus=2;
    state KeepAliveSendTimeout [parallel]
      settings: executionOrder=1
      state KeepAliveSend
      (default) -> KeepAliveSend
      KeepAliveSend -> KeepAliveSend [order 1] : after(delay_array(i)*5,msec)
          |  {OrionKeepAliveOut.data=0;
          | send(OrionKeepAliveOut);i = i + 1;}
      KeepAliveSend -> KeepAliveSend [order 2] : SendDataIn
          | {OrionAppDataOut.data=0;
          | send(OrionAppDataOut);}
    state KeepAliveRecieveTimeout [parallel]
      settings: executionOrder=2
      state KeepAlineRec
      (default) -> KeepAlineRec
      KeepAlineRec -> KeepAlineRec [order 2] : OrionKeepAliveIn
      KeepAlineRec -> KeepAlineRec [order 3] : OrionAppDataIn
  state Closed
    entry:
    connStatus=0;
  state Connecting
    entry:
    connStatus=1;
  Connected -> (junction 6) [order 2] : OrionConnRespIn
  Connected -> (junction 6) [order 3] : OrionConnReqIn
  (default) -> Closed : {i=1;}
  (junction 6) -> Closed
  Connected -> (junction 6) [order 1] : OrionConnConfIn
  KeepAlineRec -> Closed [order 1] : after(delay_array(i)*5,msec)
      | {i = i + 1;}
  Connecting -> (junction 36) [order 6] : OrionAppDataIn
  Connecting -> (junction 36) [order 5] : OrionConnReqIn
  (junction 36) -> Closed
  Connecting -> (junction 36) [order 4] : OrionConnRespIn
  Connecting -> (junction 36) [order 3] : OrionKeepAliveIn
  Closed -> Connecting : OrionConnReqIn
      | {OrionConnRespOut.data=0;
      | send(OrionConnRespOut);}
  Connecting -> Closed [order 1] : after(delay_array(i)*5,msec)
      | {i = i + 1;}
  Connecting -> Connected [order 2] : OrionConnConfIn{OrionConnConfOut.data=0;send(OrionConnConfOut);}
  data: OrionKeepAliveIn input; OrionConnConfOut output; OrionConnRespOut output; OrionKeepAliveOut output; OrionAppDataOut output; OrionAppDataIn input; OrionConnRespIn input; OrionConnReqIn input; OrionConnReqOut output size=1; connStatus output; SendDataIn local; OrionConnConfIn input; delay_array input; i local

== stateflow chart orion_casestudy_16/Slave13 ==
  settings: updateMethod=CONTINUOUS
  state Connected
    entry:
    connStatus=2;
    state KeepAliveSendTimeout [parallel]
      settings: executionOrder=1
      state KeepAliveSend
      (default) -> KeepAliveSend
      KeepAliveSend -> KeepAliveSend [order 1] : after(delay_array(i)*5,msec)
          |  {OrionKeepAliveOut.data=0;
          | send(OrionKeepAliveOut);i = i + 1;}
      KeepAliveSend -> KeepAliveSend [order 2] : SendDataIn
          | {OrionAppDataOut.data=0;
          | send(OrionAppDataOut);}
    state KeepAliveRecieveTimeout [parallel]
      settings: executionOrder=2
      state KeepAlineRec
      (default) -> KeepAlineRec
      KeepAlineRec -> KeepAlineRec [order 2] : OrionKeepAliveIn
      KeepAlineRec -> KeepAlineRec [order 3] : OrionAppDataIn
  state Closed
    entry:
    connStatus=0;
  state Connecting
    entry:
    connStatus=1;
  Connected -> (junction 6) [order 2] : OrionConnRespIn
  Connected -> (junction 6) [order 3] : OrionConnReqIn
  (default) -> Closed : {i=1;}
  (junction 6) -> Closed
  Connected -> (junction 6) [order 1] : OrionConnConfIn
  KeepAlineRec -> Closed [order 1] : after(delay_array(i)*5,msec)
      | {i = i + 1;}
  Connecting -> (junction 36) [order 6] : OrionAppDataIn
  Connecting -> (junction 36) [order 5] : OrionConnReqIn
  (junction 36) -> Closed
  Connecting -> (junction 36) [order 4] : OrionConnRespIn
  Connecting -> (junction 36) [order 3] : OrionKeepAliveIn
  Closed -> Connecting : OrionConnReqIn
      | {OrionConnRespOut.data=0;
      | send(OrionConnRespOut);}
  Connecting -> Closed [order 1] : after(delay_array(i)*5,msec)
      | {i = i + 1;}
  Connecting -> Connected [order 2] : OrionConnConfIn{OrionConnConfOut.data=0;send(OrionConnConfOut);}
  data: OrionKeepAliveIn input; OrionConnConfOut output; OrionConnRespOut output; OrionKeepAliveOut output; OrionAppDataOut output; OrionAppDataIn input; OrionConnRespIn input; OrionConnReqIn input; OrionConnReqOut output size=1; connStatus output; SendDataIn local; OrionConnConfIn input; delay_array input; i local

== stateflow chart orion_casestudy_16/DelaySwitch13 ==
  state Operation
  state Sending
  (default) -> Operation : {i=0;}
  (junction 7) -> Operation [order 2]
  Sending -> Operation : after(delay_array(i),msec)
      | {receive(inMsg);outMsg.data=0;send(outMsg);}
  Operation -> (junction 7) : inMsg{i = i + 1;}
  (junction 7) -> Sending [order 1] : [switch_array(i)==0]
  data: switch_array input; delay_array input; outMsg output; inMsg input; i local

== stateflow chart orion_casestudy_16/Slave14 ==
  settings: updateMethod=CONTINUOUS
  state Connected
    entry:
    connStatus=2;
    state KeepAliveSendTimeout [parallel]
      settings: executionOrder=1
      state KeepAliveSend
      (default) -> KeepAliveSend
      KeepAliveSend -> KeepAliveSend [order 1] : after(delay_array(i)*5,msec)
          |  {OrionKeepAliveOut.data=0;
          | send(OrionKeepAliveOut);i = i + 1;}
      KeepAliveSend -> KeepAliveSend [order 2] : SendDataIn
          | {OrionAppDataOut.data=0;
          | send(OrionAppDataOut);}
    state KeepAliveRecieveTimeout [parallel]
      settings: executionOrder=2
      state KeepAlineRec
      (default) -> KeepAlineRec
      KeepAlineRec -> KeepAlineRec [order 2] : OrionKeepAliveIn
      KeepAlineRec -> KeepAlineRec [order 3] : OrionAppDataIn
  state Closed
    entry:
    connStatus=0;
  state Connecting
    entry:
    connStatus=1;
  Connected -> (junction 6) [order 2] : OrionConnRespIn
  Connected -> (junction 6) [order 3] : OrionConnReqIn
  (default) -> Closed : {i=1;}
  (junction 6) -> Closed
  Connected -> (junction 6) [order 1] : OrionConnConfIn
  KeepAlineRec -> Closed [order 1] : after(delay_array(i)*5,msec)
      | {i = i + 1;}
  Connecting -> (junction 36) [order 6] : OrionAppDataIn
  Connecting -> (junction 36) [order 5] : OrionConnReqIn
  (junction 36) -> Closed
  Connecting -> (junction 36) [order 4] : OrionConnRespIn
  Connecting -> (junction 36) [order 3] : OrionKeepAliveIn
  Closed -> Connecting : OrionConnReqIn
      | {OrionConnRespOut.data=0;
      | send(OrionConnRespOut);}
  Connecting -> Closed [order 1] : after(delay_array(i)*5,msec)
      | {i = i + 1;}
  Connecting -> Connected [order 2] : OrionConnConfIn{OrionConnConfOut.data=0;send(OrionConnConfOut);}
  data: OrionKeepAliveIn input; OrionConnConfOut output; OrionConnRespOut output; OrionKeepAliveOut output; OrionAppDataOut output; OrionAppDataIn input; OrionConnRespIn input; OrionConnReqIn input; OrionConnReqOut output size=1; connStatus output; SendDataIn local; OrionConnConfIn input; delay_array input; i local
